simulink model "Integration_Differentiation_Project2"  (R2016b)
settings: Solver=VariableStepAuto  StartTime=0.0  StopTime=10.0  RelTol=1e-3
values from neighbouring files (symbols this model uses):
  A = 3    [Integration_Differentiation_Project2_Run.m]
  F = 2    [Integration_Differentiation_Project2_Run.m]
  Ti = 0.5    [Integration_Differentiation_Project2_Run.m]
libraries: simulink x1
settings Model: Creator=1026691  LastModifiedBy=1026691

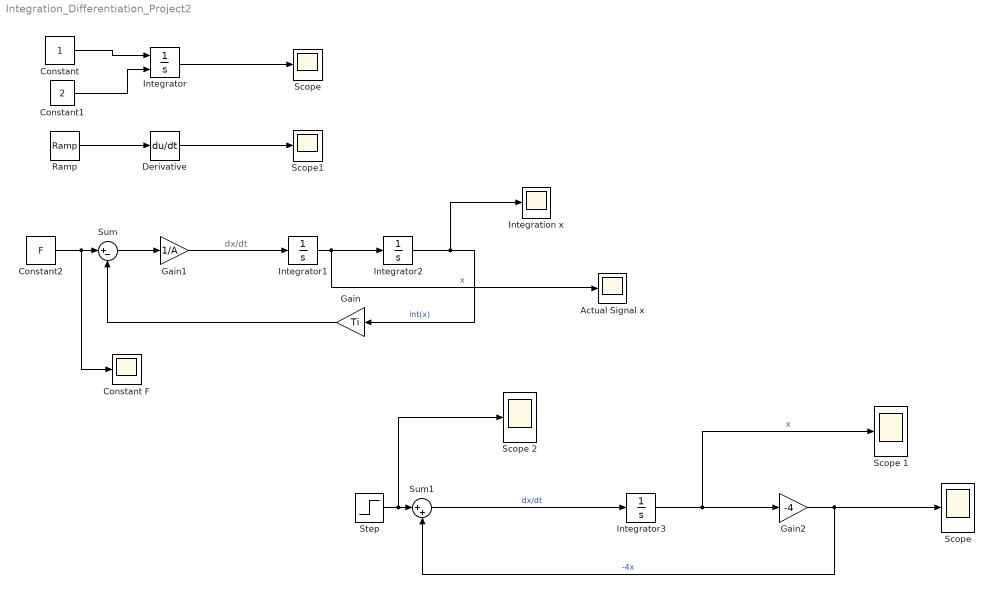
== system Integration_Differentiation_Project2 ==
  note: dx/dt
  Actual Signal x : Scope
  Constant : Constant
  "Constant F " : Scope
  Constant1 : Constant  Value=2
  Constant2 : Constant  Value=F
  Derivative : Derivative
  Gain : Gain  Gain=Ti
  Gain1 : Gain  Gain=1/A
  Gain2 : Gain  Gain=-4
  Integration x : Scope
  Integrator : Integrator  InitialConditionSource=external
  Integrator1 : Integrator
  Integrator2 : Integrator
  Integrator3 : Integrator
  Ramp : simulink/Sources/Ramp  slope=1  start=0  X0=0
  Scope : Scope
  "Scope " : Scope
  Scope 1 : Scope
  Scope 2 : Scope
  Scope1 : Scope
  Step : Step  SampleTime=0
  Sum : Sum  Inputs=|+-
  Sum1 : Sum  Inputs=|++
  wires:
  Constant/1 -> Integrator/1
  Ramp/1 -> Derivative/1
  Integrator/1 -> Scope/1
  Derivative/1 -> Scope1/1
  Constant1/1 -> Integrator/2
  Gain1/1 -> Integrator1/1
  Integrator1/1 -> Integrator2/1, Actual Signal x/1  "x"
  Integrator2/1 -> Integration x/1, Gain/1  "int(x)"
  Constant2/1 -> "Constant F "/1, Sum/1
  Gain/1 -> Sum/2
  Sum/1 -> Gain1/1
  Integrator3/1 -> Scope 1/1, Gain2/1  "x"
  Sum1/1 -> Integrator3/1  "dx/dt"
  Gain2/1 -> Sum1/2, "Scope "/1  "-4x"
  Step/1 -> Scope 2/1, Sum1/1
